simulink model "sudoku"  (R2019b)
settings: Solver=FixedStepDiscrete  StartTime=0.0  StopTime=100000000  FixedStep=1  RelTol=1e-3
PreLoadFcn:
  | variant_true_rng = false;
libraries: sudoku_lib x5
settings Model: Creator=F074018  LastModifiedBy=F074018
settings DataIOCC: ReturnWorkspaceOutputs=off
settings DebuggingCC: InheritedTsInSrcMsg=none  ArithmeticOperatorsInVariantConditions=warning
settings SFSimCC: CustomCodeUndefinedFunction=UseInterfaceOnly
settings ConfigComp: DVMode=PropertyProving  DVTestSuiteOptimization=Auto  DVDetectOutOfBounds=on

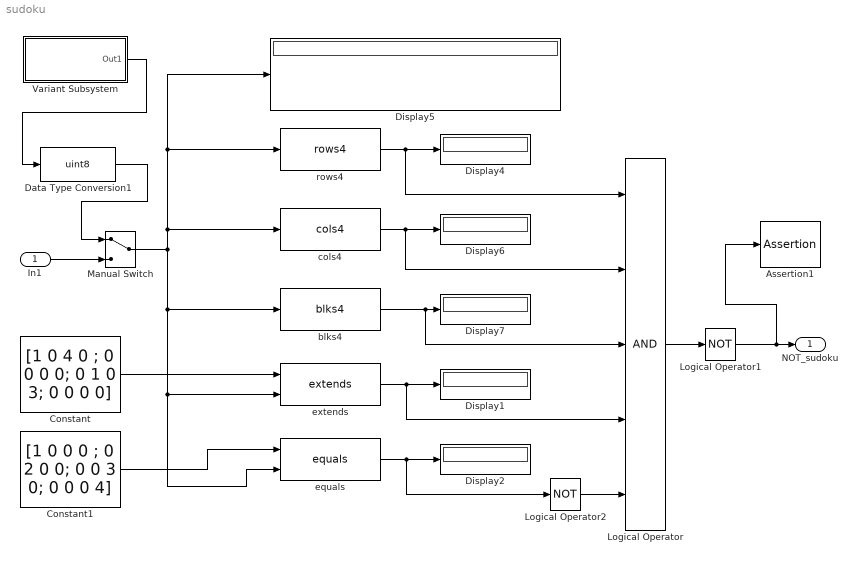
== system sudoku ==
  In1 : Inport  OutDataTypeStr=uint8  PortDimensions=[4 4]
      settings: AttributesFormatString=|
      | %<OutDataTypeStr>
      | %<PortDimensions>
  Assertion1 : Assertion
  Constant : Constant  Value=[1 0 4 0 ; 0 0 0 0; 0 1 0 3; 0 0 0 0]  OutDataTypeStr=uint8
  Constant1 : Constant  Value=[1 0 0 0 ; 0 2 0 0; 0 0 3 0; 0 0 0 4]  OutDataTypeStr=uint8
  Data Type Conversion1 : DataTypeConversion  OutDataTypeStr=uint8  RndMeth=Round
      settings: AttributesFormatString=RndMeth=%<RndMeth>
  Display{1..2,4..7} (6 alike) : Display
  Logical Operator : Logic  Inputs=5  AllPortsSameDT=off  OutDataTypeStr=boolean
  Logical Operator1 : Logic  Operator=NOT  IconShape=distinctive  AllPortsSameDT=off  OutDataTypeStr=boolean
  Logical Operator2 : Logic  Operator=NOT  IconShape=distinctive  AllPortsSameDT=off  OutDataTypeStr=boolean
  Manual Switch : ManualSwitch
  Variant Subsystem : Subsystem  Variant=on
  blks4 : sudoku_lib/blks4  SystemSampleTime=-1  Latency=0  AutoFrameSizeCalculation=off
  cols4 : sudoku_lib/cols4  SystemSampleTime=-1  Latency=0  AutoFrameSizeCalculation=off
  equals : sudoku_lib/equals  SystemSampleTime=-1  Latency=0  AutoFrameSizeCalculation=off
  extends : sudoku_lib/extends  SystemSampleTime=-1  Latency=0  AutoFrameSizeCalculation=off
  rows4 : sudoku_lib/rows4  SystemSampleTime=-1  Latency=0  AutoFrameSizeCalculation=off
  NOT_sudoku : Outport  VectorParamsAs1DForOutWhenUnconnected=off
  wires:
  rows4/1 -> Logical Operator/1, Display4/1
  cols4/1 -> Logical Operator/2, Display6/1
  blks4/1 -> Logical Operator/3, Display7/1
  Logical Operator1/1 -> Assertion1/1, NOT_sudoku/1
  Logical Operator/1 -> Logical Operator1/1
  Data Type Conversion1/1 -> Manual Switch/1
  Manual Switch/1 -> Display5/1, rows4/1, cols4/1, equals/2, extends/2, blks4/1
  In1/1 -> Manual Switch/2
  extends/1 -> Logical Operator/4, Display1/1
  Constant/1 -> extends/1
  Constant1/1 -> equals/1
  equals/1 -> Logical Operator2/1, Display2/1
  Logical Operator2/1 -> Logical Operator/5
  Variant Subsystem/1(Out1) -> Data Type Conversion1/1

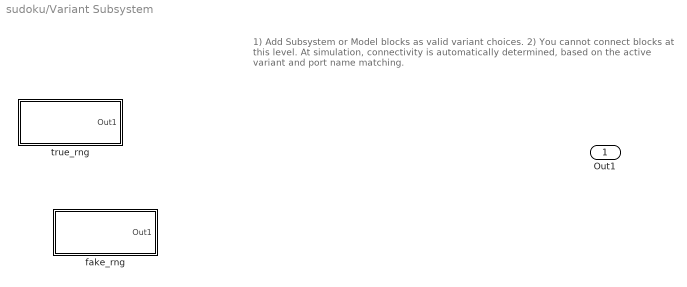
== system sudoku/Variant Subsystem ==
  note: 1) Add Subsystem or Model blocks as valid variant choices.
      | 2) You cannot connect blocks at this level. At simulation, connectivity is automatically
      | determined, based on the active variant and port name matching.
  fake_rng : Subsystem  VariantControl=variant_true_rng == false
  true_rng : Subsystem  VariantControl=(default)
  Out1 : Outport  VectorParamsAs1DForOutWhenUnconnected=off

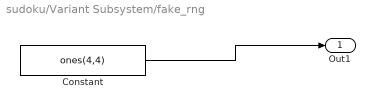
== system sudoku/Variant Subsystem/fake_rng ==
  Constant : Constant  Value=ones(4,4)
  Out1 : Outport  VectorParamsAs1DForOutWhenUnconnected=off
  wires:
  Constant/1 -> Out1/1

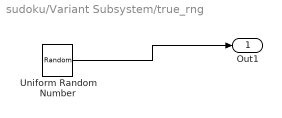
== system sudoku/Variant Subsystem/true_rng ==
  Uniform Random Number : UniformRandomNumber  Minimum=0.5 * ones(4,4)  Maximum=4.499999999 * ones(4,4)  Seed=reshape(1:16,4,4)
      settings: AttributesFormatString=|
      | Minimum=%<Minimum>
      | Maximum=%<Maximum>
  Out1 : Outport  VectorParamsAs1DForOutWhenUnconnected=off
  wires:
  Uniform Random Number/1 -> Out1/1
